simulink model "all_in_one_after"  (R2015a)
settings: Solver=FixedStepDiscrete  StartTime=0.0  StopTime=1500  FixedStep=1  RelTol=1e-3
settings Model: Creator=qiji  LastModifiedBy=qiji
settings OptimizationCC: BlockReduction=off  ConditionallyExecuteInputs=off
settings DebuggingCC: UnderspecifiedInitializationDetection=Classic  MergeDetectMultiDrivingBlocksExec=none  SolverPrmCheckMsg=warning  SingleTaskRateTransMsg=error

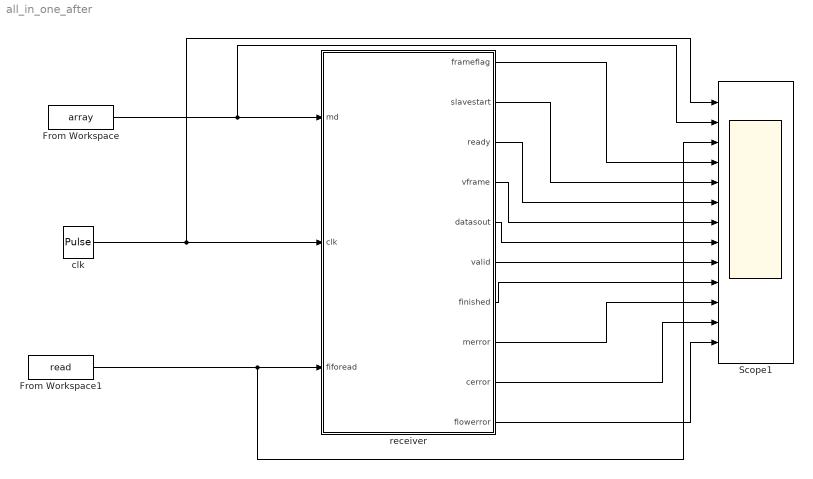
== system all_in_one_after ==
  From Workspace : FromWorkspace  VariableName=array  SampleTime=0
  From Workspace1 : FromWorkspace  VariableName=read  SampleTime=0
  Scope1 : Scope  NumInputPorts=13
      settings: YMin=-5~-5~-5~-5~-5~-5~-5~-5~-5~-5~-5~-5~-5  YMax=5~5~5~5~5~5~5~5~5~5~5~5~5
  clk : DiscretePulseGenerator  PulseType=Time based  Amplitude=true  PulseWidth=50
  receiver : Subsystem
  wires:
  clk/1 -> Scope1/1, receiver/2(clk)
  From Workspace1/1 -> Scope1/3, receiver/3(fiforead)
  From Workspace/1 -> Scope1/2, receiver/1("md ")
  receiver/1(frameflag) -> Scope1/4
  receiver/2(slavestart) -> Scope1/5
  receiver/3(ready) -> Scope1/6
  receiver/4(vframe) -> Scope1/7
  receiver/5(datasout) -> Scope1/8
  receiver/6(valid) -> Scope1/9
  receiver/7(finished) -> Scope1/10
  receiver/8(merror) -> Scope1/11
  receiver/9(cerror) -> Scope1/12
  receiver/10(flowerror) -> Scope1/13

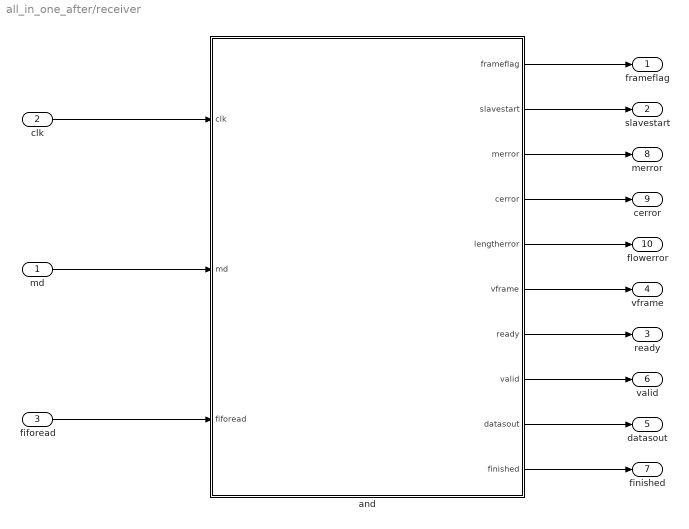
== system all_in_one_after/receiver ==
  "md " : Inport
  clk : Inport  Port=2
  fiforead : Inport  Port=3
  and : Stateflow chart  TreatAsAtomicUnit=on
  frameflag : Outport
  slavestart : Outport  Port=2
  ready : Outport  Port=3
  vframe : Outport  Port=4
  datasout : Outport  Port=5
  valid : Outport  Port=6
  finished : Outport  Port=7
  merror : Outport  Port=8
  cerror : Outport  Port=9
  flowerror : Outport  Port=10
  wires:
  clk/1 -> and/1(clk)
  "md "/1 -> and/2(md)
  fiforead/1 -> and/3(fiforead)
  and/1(frameflag) -> frameflag/1
  and/2(slavestart) -> slavestart/1
  and/3(merror) -> merror/1
  and/4(cerror) -> cerror/1
  and/5(lengtherror) -> flowerror/1
  and/6(vframe) -> vframe/1
  and/7(ready) -> ready/1
  and/8(valid) -> valid/1
  and/9(datasout) -> datasout/1
  and/10(finished) -> finished/1

== stateflow chart all_in_one_after/receiver/and ==
  settings: executeAtInitialization=1  initializeOutput=1
  state decoder [parallel]
    settings: executionOrder=4
    note: 采样4位以后，开始解码
    state s000
      en:
      masterframe=false;
      slaveframe=false;
      sample8 = uint8(0);
      du:
      s000Action();
      exit:
      s000Action();
    state s001
      s001 -> s001 [order 1] : [clk==1]
          | {
          | sample8=sample8+1;
          | sAction();
          | }
    state s100
      s100 -> s100 [order 1] : [clk==1]
          | {
          | sample8 = sample8+1;
          | sAction();
          | }
    state s101
      en:
      sample8 = sample8 + 1;
      state s01
      state s00
      s00 -> s01 [order 2] : [samples(1)==false &&samples(2)== true &&...
          | samples(3) == false &&samples(4) == true]
          | {dataRegisters(3:16) =dataRegisters(1:14);
          | dataRegisters(1:2) = [false; false];frameAction();}
      s00 -> s01 [order 1] : [samples(1)==false &&samples(2)== true &&...
          | samples(3) == true &&samples(4) == false]
          | {dataRegisters(3:16) =dataRegisters(1:14);
          | dataRegisters(1:2) = [false,true];frameAction();}
      (default) -> s00
      s00 -> s01 [order 4] : [samples(1)==true &&samples(2)== false &&...
          | samples(3) == false &&samples(4) == true]
          | {dataRegisters(3:16) = dataRegisters(1:14);
          | dataRegisters(1:2) =[true,false];frameAction();}
      s00 -> s01 [order 3] : [samples(1)==true &&samples(2)== false &&...
          | samples(3) == true &&samples(4) == false]
          | {dataRegisters(3:16) = dataRegisters(1:14);
          | dataRegisters(1:2) =  [true,true];frameAction();}
    state s01Action [function]
      (default) -> (junction 46)
      (junction 46) -> (junction 47) [order 1] : [counter8==0]
      (junction 46) -> (junction 60) [order 2] : {
          | fifowrite=false;
          | datas(1:16)=[false; false; false; false;...
          | false; false; false; false; false; false;...
          | false; false; false; false; false; false];
          | ismaster=false;
          | isslave=false;
          | }
      (junction 47) -> (junction 48)
      (junction 48) -> (junction 49) [order 1] : [total == 4]
      (junction 48) -> (junction 52) [order 2] : {total=total+1;
          | fifowrite=true;}
      (junction 49) -> (junction 50) : {total = uint8(0);}
      (junction 50) -> (junction 51) [order 1] : [xor(checkcode(2), dataRegisters(10))==true ...
          | && xor(checkcode(3), dataRegisters(11))==true ...
          | && xor(checkcode(4), dataRegisters(12))==true ...
          | && xor(checkcode(5), dataRegisters(13))==true ...
          | && xor(checkcode(6), dataRegisters(14))==true ...
          | && xor(checkcode(7), dataRegisters(15))==true ...
          | && xor(checkcode(8), dataRegisters(16))==true...
          | && xor(xor(xor(xor(xor(xor(xor(xor(checkcode(8), checkcode(7)),...
          |  checkcode(6)), checkcode(5)), checkcode(4)), checkcode(3)), ...
          | checkcode(2)), checkcode(1)), dataRegisters(9)) == true]
      (junction 50) -> (junction 54) [order 2]
      (junction 51) -> (junction 55) : {cerrorflag = true;}
      (junction 52) -> (junction 53) [order 1] : [cfl == 16]
      (junction 52) -> (junction 57) [order 2] : {cfl = cfl+1}
      (junction 53) -> (junction 56) : {overflow = true}
      (junction 55) -> (junction 54)
      (junction 54) -> (junction 59) : {
          | dataRegisters=[dataRegisters(8);...
          | dataRegisters(7); dataRegisters(6); dataRegisters(5);...
          | dataRegisters(4);dataRegisters(3);dataRegisters(2);...
          | dataRegisters(1);false; false; false; false;...
          | false; false; false; false];
          | counter8= uint8(4);
          | checkcode=[false; false; false;...
          | false; false; false; false; false];
          | ismaster=false;
          | isslave=false;
          | fifowrite=false;
          | datas=[false; false; false;...
          | false; false; false; false; false;...
          | false; false; false; false; false;...
          | false; false; false;];
          | }
      (junction 56) -> (junction 57)
      (junction 57) -> (junction 58) : {
          | datas=dataRegisters;
          | checkcode(1) = xor(xor(xor(xor(xor(xor(xor(xor(xor(xor(xor...
          | (xor(xor(xor(xor(xor(dataRegisters(15), dataRegisters(14)), ...
          | dataRegisters(13)), dataRegisters(12)), dataRegisters(11)), ...
          | dataRegisters(10)), dataRegisters(9)), dataRegisters(8)),...
          | dataRegisters(7)), dataRegisters(6)), dataRegisters(5)), ...
          | dataRegisters(4)), dataRegisters(3)), dataRegisters(2)), ...
          | dataRegisters(1)), dataRegisters(16)), checkcode(1));
          |
          | checkcode(2) = xor(xor(xor(xor(xor(xor(xor(xor(xor(xor(...
          | dataRegisters(16), dataRegisters(14)), dataRegisters(8)),...
          | dataRegisters(7)) , dataRegisters(6)), dataRegisters(5)), ...
          | dataRegisters(4)), dataRegisters(2)), dataRegisters(1)),...
          | checkcode(6)), checkcode(8));
          |
          | checkcode(3) = xor(xor(xor(xor(xor(xor(xor(xor(dataRegisters(15),...
          | dataRegisters(9)), dataRegisters(8)), dataRegisters(7)), ...
          | dataRegisters(6)), dataRegisters(5)), dataRegisters(3)), ...
          | dataRegisters(2)), checkcode(7));
          |
          | checkcode(4) = xor(xor(xor(xor(xor(xor(xor(xor(dataRegisters(14),...
          | dataRegisters(10)), dataRegisters(9)), dataRegisters(5)),...
          | dataRegisters(3)), dataRegisters(2)), dataRegisters(1)),...
          | checkcode(2)), checkcode(6));
          |
          | checkcode(5) = xor(xor(xor(xor(xor(xor(xor(xor(xor(dataRegisters(15),...
          | dataRegisters(11)), dataRegisters(10)),  dataRegisters(6)), ...
          | dataRegisters(4)), dataRegisters(3)), dataRegisters(2)),...
          | checkcode(2)), checkcode(3)), checkcode(7));
          |
          | checkcode(6) = xor(xor(xor(xor(xor(xor(xor(xor(xor(dataRegisters(16),...
          | dataRegisters(12)), dataRegisters(11)), dataRegisters(7)),...
          | dataRegisters(5)), dataRegisters(4)), dataRegisters(3)),...
          | checkcode(3)), checkcode(4)), checkcode(8));
          |
          | checkcode(7) = xor(xor(xor(xor(xor(xor(xor(xor(xor(xor(dataRegisters(16),...
          | dataRegisters(14)), dataRegisters(13)), dataRegisters(12)), ...
          | dataRegisters(7)), dataRegisters(2)), dataRegisters(1)), ...
          | checkcode(4)), checkcode(5)), checkcode(6)), checkcode(8));
          |
          | checkcode(8) = xor(xor(xor(xor(xor(xor(xor(xor(xor(xor(xor(dataRegisters(16),...
          | dataRegisters(15)), dataRegisters(13)), dataRegisters(7)), dataRegisters(6)),...
          | dataRegisters(5)), dataRegisters(4)), dataRegisters(3)), dataRegisters(1)),...
          | checkcode(5)), checkcode(7)),checkcode(8));
          |
          | ismaster=false;
          | isslave=false;
          | }
      (junction 59) -> (junction 58)
      (junction 58) -> (junction 61)
      (junction 61) -> (junction 60)
      (junction 60) -> (junction 62) : {
          | merror=false;
          | cerror=false;
          | ready=false;
          | lengtherror=false;
          | vframe=false;
          | }
    state s010
      s010 -> s010 [order 1] : [clk==1]
          | {
          | sample8 = sample8+1;
          | sAction();
          | }
    state s011
      s011 -> s011 [order 1] : [clk==1]
          | {
          | sample8 = sample8+1;
          | sAction();
          | }
    state s002s000Action [function]
      (default) -> (junction 89)
      (junction 89) -> (junction 90) [order 1] : [counter8==4]
      (junction 89) -> (junction 107) [order 2] : {
          | merror=true;
          | cerror=false;
          | ready=false;
          | ismaster=masterframe;
          | isslave=slaveframe;
          | lengtherror=false;
          | vframe=false;
          | }
      (junction 90) -> (junction 91)
      (junction 91) -> (junction 92) [order 1] : [xor(checkcode(2), dataRegisters(2))==true ...
          | && xor(checkcode(3), dataRegisters(3))==true ...
          | && xor(checkcode(4), dataRegisters(4))==true ...
          | && xor(checkcode(5), dataRegisters(5))==true ...
          | && xor(checkcode(6), dataRegisters(6))==true ...
          | && xor(checkcode(7), dataRegisters(7))==true ...
          | && xor(checkcode(8), dataRegisters(8))==true...
          | && xor(xor(xor(xor(xor(xor(xor(xor(checkcode(8), checkcode(7)),...
          |  checkcode(6)), checkcode(5)), checkcode(4)), checkcode(3)), ...
          | checkcode(2)), checkcode(1)), dataRegisters(1)) == true]
      (junction 91) -> (junction 101) [order 2] : {
          | cerror=true;
          | ready=false;
          | merror=false;
          | }
      (junction 92) -> (junction 94)
      (junction 94) -> (junction 93) [order 1] : [cerrorflag==false && overflow==false && ...
          | (cfl==1 || cfl==2 || cfl==4 || cfl==8 || cfl==16)]
      (junction 93) -> (junction 96) : {ready=true;}
      (junction 94) -> (junction 95) [order 2] : {ready = false;}
      (junction 96) -> (junction 95)
      (junction 95) -> (junction 97)
      (junction 97) -> (junction 98) [order 1] : [cerrorflag==false]
      (junction 97) -> (junction 99) [order 2] : {cerror = true;}
      (junction 98) -> (junction 100) : {cerror = false;}
      (junction 100) -> (junction 99)
      (junction 99) -> (junction 102) : {
          | checkcode=[false; false; false; false;...
          |     false; false; false; false];
          | }
      (junction 102) -> (junction 101)
      (junction 101) -> (junction 103)
      (junction 103) -> (junction 104) [order 1] : [overflow==false && (cfl==1 || ...
          | cfl==2 || cfl==4 || cfl==8 || cfl==16)]
      (junction 103) -> (junction 105) [order 2] : {lengtherror = true;}
      (junction 104) -> (junction 106) : {lengtherror = false;}
      (junction 106) -> (junction 105)
      (junction 105) -> (junction 108) : {merror = false;
          | ismaster = masterframe;
          | isslave = slaveframe;
          | vframe=true;}
      (junction 108) -> (junction 107)
      (junction 107) -> (junction 109)
    state sAction [function]
      (default) -> (junction 137) : {
          | merror=false;
          | cerror=false;
          | ismaster=false;
          | isslave=false;
          | ready=false;
          | fifowrite=false;
          | datas=[false; false; false; false;...
          |     false; false; false; false;...
          |     false; false; false; false;...
          |     false; false; false; false;];
          | lengtherror=false;
          | vframe=false;
          | }
    state frameAction [function]
      (default) -> (junction 140)
      (junction 140) -> (junction 141) [order 1] : [counter8==7]
      (junction 140) -> (junction 142) [order 2] : {counter8 = counter8+1;}
      (junction 141) -> (junction 143) : {counter8=uint8(0);}
      (junction 143) -> (junction 142)
      (junction 142) -> (junction 144) : {
          | merror=false;
          | cerror=false;
          | ismaster=false;
          | isslave=false;
          | ready=false;
          | lengtherror=false;
          | vframe=false;
          | }
    state s000Action [function]
      (default) -> (junction 152) : {
          | checkcode=[false; false; false; false;...
          |     false; false; false; false];
          | dataRegisters=[false; false; false; false;...
          |     false; false; false; false;...
          |     false; false; false; false;...
          |     false; false; false; false;];
          | samples = [false; false; false; false];
          | total= uint8(0);
          | counter8 = uint8(0);
          | merror=false;
          | cerror=false;
          | ismaster=false;
          | isslave=false;
          | ready=false;
          | fifowrite=false;
          | datas=[false; false; false; false;...
          |     false; false; false; false;...
          |     false; false; false; false;...
          |     false; false; false; false;];
          | cerrorflag=false;
          | cfl= uint8(0);
          | overflow=false;
          | lengtherror=false;
          | vframe=false;
          | }
    s00 -> s000 [order 5] : [(samples(1)==false &&...
        | samples(2)== false &&...
        | samples(3) == true &&...
        | samples(4) == true) ||...
        | ...
        | (samples(1)==false &&...
        | samples(2)== false &&...
        | samples(3) == true &&...
        | samples(4) == false) ||...
        | ...
        | (samples(1)==false &&...
        | samples(2)== false &&...
        | samples(3) == false &&...
        | samples(4) == true) ||...
        | ...
        | (samples(1)==false &&...
        | samples(2)== false &&...
        | samples(3) == false &&...
        | samples(4) == false)]
        | {
        | s002s000Action();
        | }
    s01 -> s001 : {
        | s01Action();
        | }
    s000 -> s001 : [start == true]
        | {
        | masterframe=master;
        | slaveframe=slave;
        | sample8=uint8(1);
        | }
    (default) -> s000
    s100 -> s101 [order 1] : [sample8 == 8]
        | {
        | samples = cat(1, samples(2:4), md);
        | sample8 = uint8(0);
        | sAction();
        | }
    s00 -> s000 [order 6] : {
        | merror = true;
        | cerror = false;
        | ready = false;
        | ismaster=masterframe;
        | isslave=slaveframe;
        | lengtherror=false;
        | vframe=false;
        | }
    s001 -> s010 [order 1] : [sample8 == 8]
        | {
        | samples = cat(1, samples(2:4), md);
        | sample8 = uint8(0);
        | sAction();
        | }
    s011 -> s100 [order 1] : [sample8 == 8]
        | {
        | samples = cat(1, samples(2:4), md);
        | sample8 = uint8(0);
        | sAction();
        | }
    s010 -> s011 [order 1] : [sample8==8]
        | {
        | samples = cat(1, samples(2:4), md);
        | sample8 = uint8(0);
        | sAction();
        | }
  state and [parallel]
    settings: executionOrder=7
    state start
      du:
      frameflag = ismaster && out;
    (default) -> and.start : {
        | ismaster = false;
        | out = false;
        | }
  state and1 [parallel]
    settings: executionOrder=8
    state start
      du:
      slavestart = start && slave;
    (default) -> and1.start : {
        | start = false;
        | slave = false;
        | }
  state detectMainFrame [parallel]
    settings: executionOrder=1
    state FIFO
      du:
      master = detectMainFrame(samples);
      detectMainFrame.FIFO -> detectMainFrame.FIFO : [clk==1]
          | {
          | samples  = BufferFIFO(samples, md);
          | }
    (default) -> detectMainFrame.FIFO : {
        | samples =logical(zeros(144, 1));
        | }
  state detectSlaveFrame [parallel]
    settings: executionOrder=2
    state FIFO
      du:
      slave = detectSlaveFrame(samples);
      detectSlaveFrame.FIFO -> detectSlaveFrame.FIFO : [clk==1]
          | {
          | samples  = BufferFIFO(samples, md);
          | }
    (default) -> detectSlaveFrame.FIFO : {
        | samples = logical(zeros(144,1));
        | }
  state not [parallel]
    settings: executionOrder=6
    state start
      du:
      out =~isslave;
    (default) -> not.start
  state or [parallel]
    settings: executionOrder=3
    state start
      du:
      start = master || slave;
    (default) -> or.start
  state recieveBuffer [parallel]
    settings: executionOrder=5
    state judge [function]
      (default) -> (junction 243)
      (junction 242) -> (junction 241) [order 1] : [fifowrite==true]
      (junction 243) -> (junction 242) [order 2] : [start==false]
      (junction 241) -> (junction 247)
      (junction 242) -> (junction 244) [order 2]
      (junction 243) -> (junction 258) [order 1] : [start==true]
          | {
          | tail=uint8(1);
          | head=uint8(1);
          | readtag=false;
          | valid=false;
          | finished=false;
          | datasout=zero;
          | }
      (junction 244) -> (junction 245) [order 1] : [fiforead==true]
      (junction 247) -> (junction 246) [order 1] : [tail==17]
      (junction 244) -> (junction 255) [order 2] : {
          | valid=false;
          | finished=false;
          | datasout=zero;
          | }
      (junction 245) -> (junction 248)
      (junction 247) -> (junction 251) [order 2] : {
          | fifo(:, tail)=datas;
          | tail=tail+1;
          | }
      (junction 246) -> (junction 250) : {tail=uint8(1)}
      (junction 248) -> (junction 249) [order 1] : [head==tail]
      (junction 248) -> (junction 252) [order 2] : {
          | finished=false;
          | valid=true;
          | datasout=fifo(:, head);
          | head=head+1;
          | }
      (junction 249) -> (junction 253) : {
          | head=uint8(1);
          | tail=uint8(1);
          | readtag=false;
          | finished=true;
          | valid=false;
          | datasout=zero;
          | }
      (junction 250) -> (junction 251)
      (junction 251) -> (junction 254) : {
          | valid=false;
          | finished=false;
          | datasout=zero;
          | }
      (junction 253) -> (junction 252)
      (junction 252) -> (junction 256)
      (junction 254) -> (junction 255)
      (junction 256) -> (junction 255)
      (junction 255) -> (junction 257)
      (junction 257) -> (junction 258)
    state start
      du:
      judge();
    (default) -> recieveBuffer.start : {
        | zero=[false; false;false;false;false; false; false; false;...
        |  false; false; false; false; false; false; false; false]
        | head = uint8(0);
        | tail = uint8(0);
        | valid = false;
        | finished = false;
        | }
  data: checkcode local boolean size=8; dataRegisters local boolean size=16; masterframe local boolean; slaveframe local boolean; samples local boolean size=4; total local uint8; counter8 local uint8; sample8 local uint8; cerrorflag local boolean; overflow local boolean; cfl local uint8; A function_input boolean size=144; c function_input boolean; r function_output boolean size=144; A function_input boolean size=144; r function_output boolean; samples local boolean size=144; m1front local boolean =0; m2front local boolean =0; m3front local boolean =0; m4front local boolean =0; m5front local boolean =0; m6front local boolean =0; m7front local boolean =0; m8front local boolean =0; m9front local boolean =0; m1back local boolean =0; m2back local boolean =0; m3back local boolean =0; m4back local boolean =0; m5back local boolean =0; m6back local boolean =0; m7back local boolean =0; m8back local boolean =0; m9back local boolean =0; A function_input boolean size=144; c function_input boolean; r function_output boolean size=144; A function_input boolean size=144; r function_output boolean; samples local boolean size=144; s1front local boolean =0; s2front local boolean =0; s3front local boolean =0; s4front local boolean =0; s5front local boolean =0; s6front local boolean =0; s7front local boolean =0; s8front local boolean =0; s9front local boolean =0; s1back local boolean =0; s2back local boolean =0; s3back local boolean =0; s4back local boolean =0; s5back local boolean =0; s6back local boolean =0; s7back local boolean =0; s8back local boolean =0; s9back local boolean =0; head local uint8; tail local uint8; readtag local boolean; zero local boolean size=16 =[0,0,0,0,0,0,0,0,0,0,0,0,0,0,0,0]; fifo local boolean size=16,16; frameflag output boolean; slavestart output boolean; merror output boolean; cerror output boolean; lengtherror output boolean; ismaster local boolean; isslave local boolean; vframe output boolean; ready output boolean; fifowrite local boolean; datas local boolean size=16; clk input boolean; md input boolean; master local boolean; slave local boolean; out local boolean; start local boolean; fiforead input boolean; valid output boolean; datasout output boolean size=16; finished output boolean
  data checkcode settings: description=存放checkcode
  data dataRegisters settings: description=存放manchester解码后的数据
  data masterframe settings: description=the symbol of master frame
  data slaveframe settings: description=the symbol of slave frame
  data samples settings: description=store 4 bits sample value
  data total settings: description=add 1 per 16 bit
  data counter8 settings: description=the number of data in dataRegisters
  data sample8 settings: description=sample the value per 8 cycle
  data cerrorflag settings: description=标识符：标识校验码错误；‘1’表示有校验码错误，‘0’表示没有检验码错误
  data overflow settings: description=溢出标识位：‘1’表示有溢出，‘0’表示没有溢出
  data head settings: description=address of the quence head
  data tail settings: description=address of quence tail
  data readtag settings: description=the sample of reading data
  data frameflag settings: description=out
  data slavestart settings: description=out
  data merror settings: description=out
  data cerror settings: description=out
  data lengtherror settings: description=out
  data vframe settings: description=out
  data ready settings: description=out
  data clk settings: description=in
  data md settings: description=in
  data fiforead settings: description=in
  data valid settings: description=out
  data datasout settings: description=out
  data finished settings: description=out
  function r = BufferFIFO(A, c):
    | function r = BufferFIFO(A, c)
    | A(2:144) = A(1:143);
    | A(1) = c;
    | r = A;
  function r = detectMainFrame(A):
    | function r = detectMainFrame(A)
    | % start
    | % case samples(143 downto 136) is
    | %		       when"11111111"|"11111110"|"11111101"|"11111011"|"11110111"|"11101111"|"11011111"|"10111111"|"01111111"|"00111111"|"11111100"|"01111110"|"00111100"=>%
    | %			        m1front<='1';
    | %			    when others=>
    | %			        m1front<='0';
    | %		  end case;
    | %		  --检测帧起始符的后半部分
    | %		  case samples(135 downto 128)  is
    | %		       when "00000000"|"00000001"|"00000010"|"00000100"|"00001000"|"00010000"|"00100000"|"01000000"|"10000000"|"11000000"|"00000011"|"10000001"|"11000011"=>
    | %			        m1back<='1';
    | %			    when others=>
    | %			        m1back<='0';
    | %		  end case;
    | if (A(137)==1 && A(138)==1 && A(139)==1&& A(140)==1&& A(141)==1&& A(142)==1&& A(143)==1&& A(144)==1) || ...
    |     (A(137)==1 && A(138)==0 && A(139)==1&& A(140)==1&& A(141)==1&& A(142)==1&& A(143)==1&& A(144)==1) || ...
    |     (A(137)==1 && A(138)==1 && A(139)==0&& A(140)==1&& A(141)==1&& A(142)==1&& A(143)==1&& A(144)==1) || ...
    |     (A(137)==1 && A(138)==1 && A(139)==1&& A(140)==0&& A(141)==1&& A(142)==1&& A(143)==1&& A(144)==1) || ...
    |     (A(137)==1 && A(138)==1 && A(139)==1&& A(140)==1&& A(141)==0&& A(142)==1&& A(143)==1&& A(144)==1) || ...
    |     (A(137)==1 && A(138)==1 && A(139)==1&& A(140)==1&& A(141)==1&& A(142)==0&& A(143)==1&& A(144)==1) || ...
    |     (A(137)==1 && A(138)==1 && A(139)==1&& A(140)==1&& A(141)==1&& A(142)==1&& A(143)==0&& A(144)==1) || ...
    |     (A(137)==1 && A(138)==1 && A(139)==1&& A(140)==1&& A(141)==1&& A(142)==1&& A(143)==1&& A(144)==0) || ...
    |     (A(137)==1 && A(138)==1 && A(139)==1&& A(140)==1&& A(141)==1&& A(142)==1&& A(143)==0&& A(144)==0) || ...
    |     (A(137)==0 && A(138)==0 && A(139)==1&& A(140)==1&& A(141)==1&& A(142)==1&& A(143)==1&& A(144)==1) || ...
    |     (A(137)==0 && A(138)==1 && A(139)==1&& A(140)==1&& A(141)==1&& A(142)==1&& A(143)==1&& A(144)==0) || ...
    |     (A(137)==0 && A(138)==0 && A(139)==1&& A(140)==1&& A(141)==1&& A(142)==1&& A(143)==0&& A(144)==0)
    |     m1front = true;
    | else
    |     m1front = false;
    | end
    | if (A(129)==0 && A(130)==0 && A(131)==0 && A(132)==0 && A(133)==0 && A(134)==0&& A(135)==0&& A(136)==0) || ...
    |         (A(129)==0 && A(130)==0 && A(131)==0 && A(132)==0 && A(133)==0 && A(134)==0&& A(135)==0&& A(136)==1) || ...
    |         (A(129)==0 && A(130)==0 && A(131)==0 && A(132)==0 && A(133)==0 && A(134)==0&& A(135)==1&& A(136)==0) || ...
    |         (A(129)==0 && A(130)==0 && A(131)==0 && A(132)==0 && A(133)==0 && A(134)==1&& A(135)==0&& A(136)==0) || ...
    |         (A(129)==0 && A(130)==0 && A(131)==0 && A(132)==0 && A(133)==1 && A(134)==0&& A(135)==0&& A(136)==0) || ...
    |         (A(129)==0 && A(130)==0 && A(131)==0 && A(132)==1 && A(133)==0 && A(134)==0&& A(135)==0&& A(136)==0) || ...
    |         (A(129)==0 && A(130)==0 && A(131)==1 && A(132)==0 && A(133)==0 && A(134)==0&& A(135)==0&& A(136)==0) || ...
    |         (A(129)==0 && A(130)==1 && A(131)==0 && A(132)==0 && A(133)==0 && A(134)==0&& A(135)==0&& A(136)==0) || ...
    |         (A(129)==1 && A(130)==0 && A(131)==0 && A(132)==0 && A(133)==0 && A(134)==0&& A(135)==0&& A(136)==0) || ...
    |         (A(129)==1 && A(130)==1 && A(131)==0 && A(132)==0 && A(133)==0 && A(134)==0&& A(135)==0&& A(136)==0) || ...
    |         (A(129)==0 && A(130)==0 && A(131)==0 && A(132)==0 && A(133)==0 && A(134)==0&& A(135)==1&& A(136)==1) || ...
    |         (A(129)==1 && A(130)==0 && A(131)==0 && A(132)==0 && A(133)==0 && A(134)==0&& A(135)==0&& A(136)==1) || ...
    |         (A(129)==1 && A(130)==1 && A(131)==0 && A(132)==0 && A(133)==0 && A(134)==0&& A(135)==1&& A(136)==1)
    |     m1back = true;
    | else
    |     m1back = false;
    | end
    | %%%%%%%%%%%%%%%%%%%%%%%%%%%%%%%%%%%%%%%%%%%%%%%%%%%%%%%%%%%%%%%%%%%%%%%%%%%%%%%%%%%%%%%%%%%%%%%%%%%%%%%%%%%%%%%%%%%%%%%%%%%%%%%%%%%%%%%%%%%%%%%%%%%%%%
    | if A(124) == 1
    |     m2front = true;
    | else
    |     m2front = false;
    | end
    | if A(116) == 1
    |     m2back = true;
    | else
    |     m2back = false;
    | end
    | if A(108) == 0
    |     m3front = true;
    | else
    |     m3front = false;
    | end
    | if A(100) == 0
    |     m3back = true;
    | else
    |     m3back = false;
    | end
    | if A(92) == 0
    |     m4front = true;
    | else
    |     m4front = false;
    | end
    | if A(84) == 1
    |     m4back = true;
    | else
    |     m4back = false;
    | end
    | if A(76) == 1
    |     m5front = true ;
    | else
    |     m5front = false;
    | end
    | if A(68) == 1
    |     m5back = true;
    | else
    |     m5back = false;
    | end
    | if A(60) == 0
    |     m6front = true;
    | else
    |     m6front = false;
    | end
    | if A(52) == 0
    |     m6back = true;
    | else
    |     m6back = false;
    | end
    | if A(44) == 0
    |     m7front = true;
    | else
    |     m7front = false;
    | end
    | if A(36) == 1
    |     m7back = true;
    | else
    |     m7back = false;
    | end
    | if A(28) == 0
    |     m8front = true;
    | else
    |     m8front = false;
    | end
    | if A(20) == 1
    |     m8back = true;
    | else
    |     m8back = false;
    | end
    | if A(12) == 0
    |     m9front = true;
    | else
    |     m9front = false;
    | end
    | if A(4) == 1
    |     m9back = true;
    | else
    |     m9back = false;
    | end
    | r = m1front && m2front && m3front && m4front && m5front && m6front && m7front && m8front && m9front && m1back && m2back && m3back && m4back && m5back && m6back && m7back && m8back && m9back;
  function r = BufferFIFO(A, c):
    | function r = BufferFIFO(A, c)
    | A(2:144) = A(1:143);
    | A(1) = c;
    | r = A;
  function r = detectSlaveFrame(A):
    | function r = detectSlaveFrame(A)
    | % start DetectSlave slave%%%%%%%%%%%%%%%%%%%%%%%%%%%%%%%%%%%%%%%%%%%%%%%%%%%%%%%%%%%%%%%%%%%%%%%%%%%%%%%%%%%%%%%%%%%%%%%%%%%%%%%%
    | if (A(137)==1 && A(138)==1 && A(139)==1&& A(140)==1&& A(141)==1&& A(142)==1&& A(143)==1&& A(144)==1) || ...
    |     (A(137)==1 && A(138)==0 && A(139)==1&& A(140)==1&& A(141)==1&& A(142)==1&& A(143)==1&& A(144)==1) || ...
    |     (A(137)==1 && A(138)==1 && A(139)==0&& A(140)==1&& A(141)==1&& A(142)==1&& A(143)==1&& A(144)==1) || ...
    |     (A(137)==1 && A(138)==1 && A(139)==1&& A(140)==0&& A(141)==1&& A(142)==1&& A(143)==1&& A(144)==1) || ...
    |     (A(137)==1 && A(138)==1 && A(139)==1&& A(140)==1&& A(141)==0&& A(142)==1&& A(143)==1&& A(144)==1) || ...
    |     (A(137)==1 && A(138)==1 && A(139)==1&& A(140)==1&& A(141)==1&& A(142)==0&& A(143)==1&& A(144)==1) || ...
    |     (A(137)==1 && A(138)==1 && A(139)==1&& A(140)==1&& A(141)==1&& A(142)==1&& A(143)==0&& A(144)==1) || ...
    |     (A(137)==1 && A(138)==1 && A(139)==1&& A(140)==1&& A(141)==1&& A(142)==1&& A(143)==1&& A(144)==0) || ...
    |     (A(137)==1 && A(138)==1 && A(139)==1&& A(140)==1&& A(141)==1&& A(142)==1&& A(143)==0&& A(144)==0) || ...
    |     (A(137)==0 && A(138)==0 && A(139)==1&& A(140)==1&& A(141)==1&& A(142)==1&& A(143)==1&& A(144)==1) || ...
    |     (A(137)==0 && A(138)==1 && A(139)==1&& A(140)==1&& A(141)==1&& A(142)==1&& A(143)==1&& A(144)==0) || ...
    |     (A(137)==0 && A(138)==0 && A(139)==1&& A(140)==1&& A(141)==1&& A(142)==1&& A(143)==0&& A(144)==0)
    |     s1front = true;
    | else
    |     s1front = false;
    | end
    | if (A(129)==0 && A(130)==0 && A(131)==0 && A(132)==0 && A(133)==0 && A(134)==0&& A(135)==0&& A(136)==0) || ...
    |         (A(129)==0 && A(130)==0 && A(131)==0 && A(132)==0 && A(133)==0 && A(134)==0&& A(135)==0&& A(136)==1) || ...
    |         (A(129)==0 && A(130)==0 && A(131)==0 && A(132)==0 && A(133)==0 && A(134)==0&& A(135)==1&& A(136)==0) || ...
    |         (A(129)==0 && A(130)==0 && A(131)==0 && A(132)==0 && A(133)==0 && A(134)==1&& A(135)==0&& A(136)==0) || ...
    |         (A(129)==0 && A(130)==0 && A(131)==0 && A(132)==0 && A(133)==1 && A(134)==0&& A(135)==0&& A(136)==0) || ...
    |         (A(129)==0 && A(130)==0 && A(131)==0 && A(132)==1 && A(133)==0 && A(134)==0&& A(135)==0&& A(136)==0) || ...
    |         (A(129)==0 && A(130)==0 && A(131)==1 && A(132)==0 && A(133)==0 && A(134)==0&& A(135)==0&& A(136)==0) || ...
    |         (A(129)==0 && A(130)==1 && A(131)==0 && A(132)==0 && A(133)==0 && A(134)==0&& A(135)==0&& A(136)==0) || ...
    |         (A(129)==1 && A(130)==0 && A(131)==0 && A(132)==0 && A(133)==0 && A(134)==0&& A(135)==0&& A(136)==0) || ...
    |         (A(129)==1 && A(130)==1 && A(131)==0 && A(132)==0 && A(133)==0 && A(134)==0&& A(135)==0&& A(136)==0) || ...
    |         (A(129)==0 && A(130)==0 && A(131)==0 && A(132)==0 && A(133)==0 && A(134)==0&& A(135)==1&& A(136)==1) || ...
    |         (A(129)==1 && A(130)==0 && A(131)==0 && A(132)==0 && A(133)==0 && A(134)==0&& A(135)==0&& A(136)==1) || ...
    |         (A(129)==1 && A(130)==1 && A(131)==0 && A(132)==0 && A(133)==0 && A(134)==0&& A(135)==1&& A(136)==1)
    |     s1back = true;
    | else
    |     s1back = false;
    | end
    | %%%%%%%%%%%%%%%%%%%%%%%%%%%%%%%%%%%%%%%%%%%%%%%%%%%%%%%%%%%%%%%%%%%%%%%%%%%%%%%%%%%%%%%%%%%%%%%%%%%%%%%%%%%%%%%%%%%%%%%%%%%%%%%%%%%%%%%%%%%%%
    | if A(124) == 1
    |     s2front = true;
    | else
    |     s2front = false;
    | end
    | if A(116) == 0
    |     s2back = true;
    | else
    |     s2back = false;
    | end
    | if A(108) == 1
    |     s3front = true;
    | else
    |     s3front = false;
    | end
    | if A(100) == 0
    |     s3back = true;
    | else
    |     s3back = false;
    | end
    | if A(92) == 1
    |     s4front = true;
    | else
    |     s4front = false;
    | end
    | if A(84) == 0
    |     s4back = true;
    | else
    |     s4back = false;
    | end
    | if A(76) == 0
    |     s5front = true ;
    | else
    |     s5front = false;
    | end
    | if A(68) == 0
    |     s5back = true;
    | else
    |     s5back = false;
    | end
    | if A(60) == 1
    |     s6front = true;
    | else
    |     s6front = false;
    | end
    | if A(52) == 1
    |     s6back = true;
    | else
    |     s6back = false;
    | end
    | if A(44) == 1
    |     s7front = true;
    | else
    |     s7front = false;
    | end
    | if A(36) == 0
    |     s7back = true;
    | else
    |     s7back = false;
    | end
    | if A(28) == 0
    |     s8front = true;
    | else
    |     s8front = false;
    | end
    | if A(20) == 0
    |     s8back = true;
    | else
    |     s8back = false;
    | end
    | if A(12) == 1
    |     s9front = true;
    | else
    |     s9front = false;
    | end
    | if A(4) == 1
    |     s9back = true;
    | else
    |     s9back = false;
    | end
    | r = s1front && s2front && s3front && s4front && s5front && s6front && s7front && s8front && s9front && s1back && s2back && s3back && s4back && s5back && s6back && s7back && s8back && s9back;
